simulink model "sf_msg_priority_queue_server"  (R2017b)
settings: Solver=ode45  StartTime=0.0  StopTime=50  RelTol=1e-3  EnableMultiTasking=on
PreLoadFcn:
  | queueLength = 10;
CloseFcn:
  | delete(findall(0, 'type', 'figure', 'tag', 'SF_SERVER'))
  | clear('queueLength')
settings Model: ExtModeAutoUpdateStatusClock=off  Creator=The MathWorks, Inc.  LastModifiedBy=The MathWorks, Inc.
settings DataIOCC: LimitDataPoints=on  SaveFormat=Array  SignalLoggingName=logsOut
settings OptimizationCC: ExpressionDepthLimit=2147483647  InitFltsAndDblsToZero=on  EfficientMapNaN2IntZero=off  LifeSpan=inf
settings DebuggingCC: UnderspecifiedInitializationDetection=Classic  MergeDetectMultiDrivingBlocksExec=none  CheckExecutionContextPreStartOutputMsg=on  CheckExecutionContextRuntimeOutputMsg=on  SignalResolutionControl=TryResolveAllWithWarning  MultiTaskDSMMsg=warning  MultiTaskCondExecSysMsg=none  FcnCallInpInsideContextMsg=warning  AllowSymbolicDim=off  StateNameClashWarn=warning  SFUnexpectedBacktrackingDiag=warning  SFNoUnconditionalDefaultTransitionDiag=warning  SFExecutionAtInitializationDiag=none
settings HardwareCC: ProdBitPerPointer=32  ProdBitPerSizeT=32  ProdBitPerPtrDiffT=32  ProdLargestAtomicFloat=None  ProdIntDivRoundTo=Undefined  ProdEndianess=Unspecified  ProdWordSize=32  ProdHWDeviceType=32-bit Generic  TargetUnknown=on
settings ModelReferenceCC: PropagateSignalLabelsOutOfModel=off
settings SFSimCC: SimParseCustomCode=off
settings CodeAppCC: StateflowObjectComments=on
settings GRTTargetCC: TargetLangStandard=C89/C90 (ANSI)  GeneratePreprocessorConditionals=Disable all  CombineOutputUpdateFcns=off  GRTInterface=on
settings ConfigComp: CovMetricSettings=dcmtr  CovHtmlReporting=on  CovSaveCumulativeToWorkspaceVar=on  CovSaveSingleToWorkspaceVar=on  CovExternalEMLEnable=off  CovSFcnEnable=off

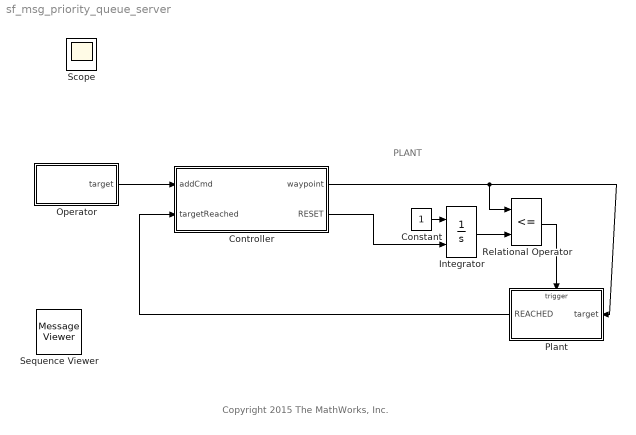
== system sf_msg_priority_queue_server ==
  note: PLANT
  note: Copyright 2015 The MathWorks, Inc.
  Constant : Constant
  Controller : Stateflow chart  TreatAsAtomicUnit=on
  Integrator : Integrator  ExternalReset=either
  Operator : Stateflow chart  TreatAsAtomicUnit=on
  Plant : Stateflow chart  TreatAsAtomicUnit=on
  Relational Operator : RelationalOperator  Operator=<=  OutDataTypeStr=boolean  RndMeth=Nearest
  Sequence Viewer : MessageViewer
  Scope : Scope
  wires:
  Operator/1(target) -> Controller/1(addCmd)
  Controller/2(RESET) -> Integrator/2
  Constant/1 -> Integrator/1
  Integrator/1 -> Relational Operator/2
  Plant/1(REACHED) -> Controller/2(targetReached)
  Controller/1(waypoint) -> Relational Operator/1, Plant/1(target)
  Relational Operator/1 -> Plant/Trigger

== stateflow chart sf_msg_priority_queue_server/Plant ==
  (default) -> (junction 3) : EVENT {REACHED.data = target; send(REACHED);}
  data: REACHED output; target input size=1
  events: EVENT input RISING_EDGE_EVENT

== stateflow chart sf_msg_priority_queue_server/Operator ==
  state Send
  state Pause
    ex:
    coder.extrinsic('pause');
    pause(.1);
  (default) -> Send
  Pause -> Send : after(0.5,sec)
  Send -> (junction 24) : {x = floor(rand().*20);}
  (junction 36) -> Pause
  (junction 24) -> (junction 25) [order 1] : [x>=19]{target.data = 5;}
  (junction 25) -> (junction 27)
  (junction 24) -> (junction 26) [order 2]
  (junction 26) -> (junction 27) [order 1] : [x>=18]{target.data = 4;}
  (junction 26) -> (junction 28) [order 2]
  (junction 27) -> (junction 29)
  (junction 28) -> (junction 29) [order 1] : [x>=17]{target.data = 3;}
  (junction 28) -> (junction 30) [order 2]
  (junction 29) -> (junction 31)
  (junction 30) -> (junction 31) [order 1] : [x>=15]{target.data = 2;}
  (junction 30) -> (junction 32) [order 2]
  (junction 31) -> (junction 33)
  (junction 32) -> (junction 33) [order 1] : [x>=14]{target.data = 1;}
  (junction 32) -> (junction 35) [order 2]
  (junction 33) -> (junction 34) : {send(target);}
  (junction 35) -> (junction 34)
  (junction 34) -> (junction 36)
  data: x local double size=1; target output double size=1

== stateflow chart sf_msg_priority_queue_server/Controller ==
  state Idle
  state Busy
  (default) -> Idle
  Idle -> Busy : addCmd
      | {
      | send(RESET);
      | waypoint = addCmd.data;
      | }
  Busy -> Idle : targetReached
  data: waypoint output size=1; addCmd input size=1; targetReached input
  events: RESET output EITHER_EDGE_EVENT
